simulink model "echo"  (R2024a)
settings: Solver=VariableStepAuto  StartTime=0.0  StopTime=20  RelTol=1e-3
libraries: hdlsllib x2
settings Model: Creator=fermata  LastModifiedBy=fermata

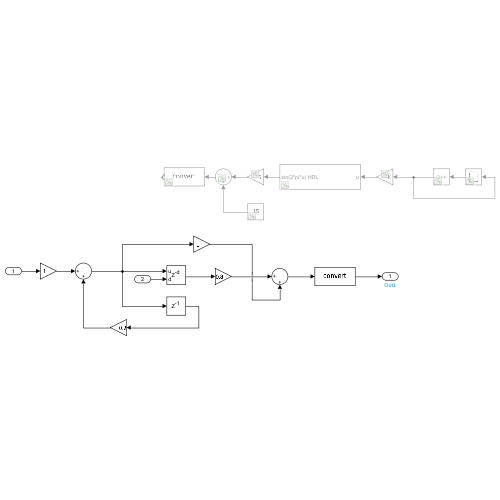
[thumbnail: Simulink's stored preview of the top-level diagram]
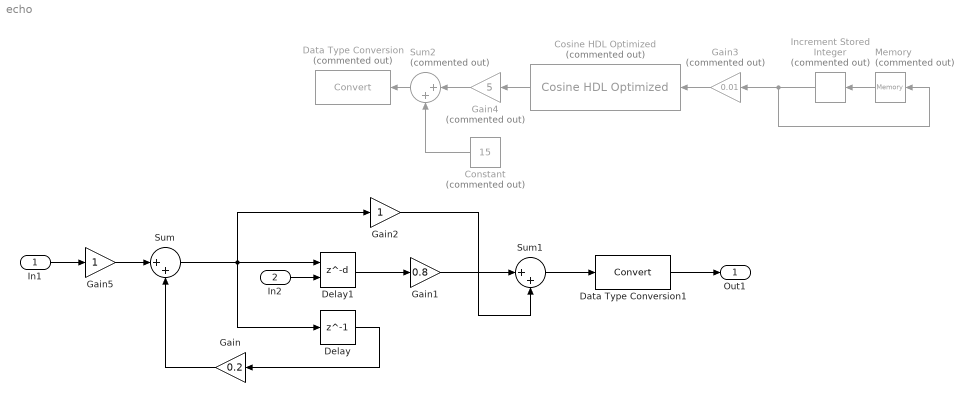
== system echo ==
  In1 : Inport  OutDataTypeStr=int16
  In2 : Inport  Port=2
  Constant : Constant  Commented=on  Value=15
  Cosine HDL Optimized : hdlsllib/Lookup Tables/Cosine HDL Optimized  Commented=on  OutputFormula=sin(2*pi*u)  NumDataPoints=1024  TableDataTypeStr=fixdt(0,16,15)  SimulateLUTROMDelay=off
  Data Type Conversion : DataTypeConversion  Commented=on  RndMeth=Round  SaturateOnIntegerOverflow=off
  Data Type Conversion1 : DataTypeConversion  SaturateOnIntegerOverflow=off  RndMeth=Floor
  Delay : Delay  DelayLength=1  InitialCondition=0
  Delay1 : Delay  DelayLengthSource=Input port  DelayLength=1  DelayLengthUpperLimit=1024  InitialCondition=0
      settings: InputPortMap=u0,p1
  Gain : Gain  Gain=0.2  OutDataTypeStr=Inherit: Inherit via back propagation  RndMeth=Simplest  SaturateOnIntegerOverflow=on
  Gain1 : Gain  Gain=0.8
  Gain2 : Gain
  Gain3 : Gain  Commented=on  Gain=0.01
  Gain4 : Gain  Commented=on  Gain=5
  Gain5 : Gain
  Increment Stored Integer : hdlsllib/Math Operations/Increment Stored Integer  Commented=on
  Memory : Memory  Commented=on  InheritSampleTime=on
  Sum : Sum  Inputs=|++
  Sum1 : Sum  Inputs=|++
  Sum2 : Sum  Commented=on  Inputs=|++
  Out1 : Outport  OutDataTypeStr=int16
  wires:
  Increment Stored Integer/1 -> Memory/1, Gain3/1
  Cosine HDL Optimized/1 -> Gain4/1
  Gain/1 -> Sum/2
  Constant/1 -> Sum2/2
  Memory/1 -> Increment Stored Integer/1
  Gain4/1 -> Sum2/1
  Delay/1 -> Gain/1
  Sum2/1 -> Data Type Conversion/1
  Gain3/1 -> Cosine HDL Optimized/1
  Gain2/1 -> Sum1/2
  Gain1/1 -> Sum1/1
  Sum1/1 -> Data Type Conversion1/1
  In1/1 -> Gain5/1
  Sum/1 -> Gain2/1, Delay/1, Delay1/1
  Delay1/1 -> Gain1/1
  In2/1 -> Delay1/2
  Data Type Conversion1/1 -> Out1/1
  Gain5/1 -> Sum/1
